simulink model "multi__micro1primarysecondarynn"  (R2015a)
settings: Solver=ode23tb  StartTime=0.0  StopTime=2
model workspace: external: MAT-File D:\google drive\project\nn1\matla.mat (data not in the file)
undefined symbols (not defined in the file): cf, gam, gamp, k1, k2, k3, k5, Lc, lf, mp1, mp2, Mu, nq1, nq2, rc, sig, sigp, td, wn
libraries: powerlib x115, powerlib_meascontrol x32, powerlib_extras x2
(part 1 of 3)
settings Model: Creator=David  LastModifiedBy=David
settings SolverCC: ZeroCrossControl=DisableAll  ZeroCrossAlgorithm=Adaptive  AlgebraicLoopSolver=LineSearch
settings DataIOCC: LimitDataPoints=off  SaveFormat=StructureWithTime  SaveOutput=off  SignalLogging=off  SaveTime=off
settings OptimizationCC: EfficientMapNaN2IntZero=off  SimCompilerOptimization=on
settings DebuggingCC: MaxConsecutiveZCsMsg=none
settings HardwareCC: TargetLongLongMode=on  TargetIntDivRoundTo=Zero  TargetEndianess=LittleEndian  TargetHWDeviceType=MATLAB Host  ProdEqTarget=off
settings CodeAppCC: MaxIdLength=128
settings GRTTargetCC: CombineOutputUpdateFcns=off  GRTInterface=on  RTWCAPISignals=on

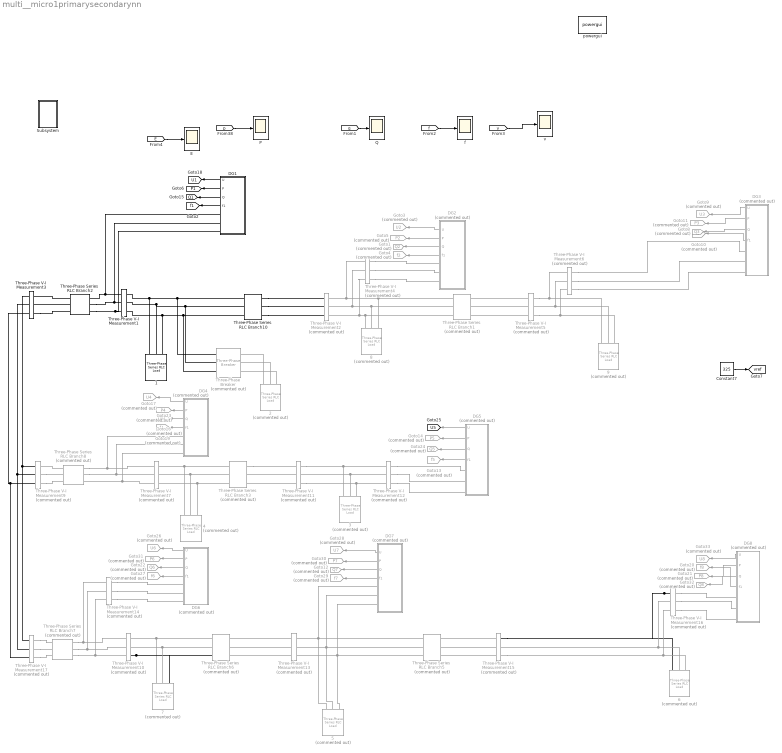
== system multi__micro1primarysecondarynn ==
  "  1" : powerlib/Elements/Three-Phase Series RLC Load  LConnTagsString=A|B|C  Configuration=Y (grounded)  NominalVoltage=vrms  NominalFrequency=50  ActivePower=18.5e3  InductivePower=14e3  CapacitivePower=0  Measurements=None  LoadType=constant Z
  "  2" : powerlib/Elements/Three-Phase Series RLC Load  Commented=on  LConnTagsString=A|B|C  Configuration=Y (grounded)  NominalVoltage=vrms  NominalFrequency=50  ActivePower=18.5e3  InductivePower=14e3  CapacitivePower=0  Measurements=None  LoadType=constant Z
  "  3" : powerlib/Elements/Three-Phase Series RLC Load  Commented=on  LConnTagsString=A|B|C  Configuration=Y (grounded)  NominalVoltage=vrms  NominalFrequency=50  ActivePower=16e3  InductivePower=11e3  CapacitivePower=0  Measurements=None  LoadType=constant Z
  "  4" : powerlib/Elements/Three-Phase Series RLC Load  Commented=on  LConnTagsString=A|B|C  Configuration=Y (grounded)  NominalVoltage=vrms  NominalFrequency=50  ActivePower=18.5e3  InductivePower=14e3  CapacitivePower=0  Measurements=None  LoadType=constant Z
  "  5" : powerlib/Elements/Three-Phase Series RLC Load  Commented=on  LConnTagsString=A|B|C  Configuration=Y (grounded)  NominalVoltage=vrms  NominalFrequency=50  ActivePower=15.3e3  InductivePower=10e3  CapacitivePower=0  Measurements=None  LoadType=constant Z
  "  6" : powerlib/Elements/Three-Phase Series RLC Load  Commented=on  LConnTagsString=A|B|C  Configuration=Y (grounded)  NominalVoltage=vrms  NominalFrequency=50  ActivePower=15.6e3  InductivePower=9.6e3  CapacitivePower=0  Measurements=None  LoadType=constant Z
  "  7" : powerlib/Elements/Three-Phase Series RLC Load  Commented=on  LConnTagsString=A|B|C  Configuration=Y (grounded)  NominalVoltage=vrms  NominalFrequency=50  ActivePower=20e3  InductivePower=15e3  CapacitivePower=0  Measurements=None  LoadType=constant Z
  "  8" : powerlib/Elements/Three-Phase Series RLC Load  Commented=on  LConnTagsString=A|B|C  Configuration=Y (grounded)  NominalVoltage=vrms  NominalFrequency=50  ActivePower=15e3  InductivePower=12e3  CapacitivePower=0  Measurements=None  LoadType=constant Z
  "  9" : powerlib/Elements/Three-Phase Series RLC Load  Commented=on  LConnTagsString=A|B|C  Configuration=Y (grounded)  NominalVoltage=vrms  NominalFrequency=50  ActivePower=12e3  InductivePower=8e3  CapacitivePower=0  Measurements=None  LoadType=constant Z
  Constant7 : Constant  Value=325
  DG1 : Subsystem
  DG2 : Subsystem  Commented=on
  DG3 : Subsystem  Commented=on
  DG4 : Subsystem  Commented=on
  DG5 : Subsystem  Commented=on
  DG6 : Subsystem  Commented=on
  DG7 : Subsystem  Commented=on
  DG8 : Subsystem  Commented=on
  E : Scope
      settings: TimeRange=0.03351610580764283  YMin=-1.5  YMax=-0.1  SaveName=E
  Goto1 : Goto  Commented=on  GotoTag=Q2  TagVisibility=global
  Goto10 : Goto  Commented=on  GotoTag=f3  TagVisibility=global
  Goto11 : Goto  Commented=on  GotoTag=P3  TagVisibility=global
  Goto12 : Goto  Commented=on  GotoTag=Q7  TagVisibility=global
  Goto13 : Goto  Commented=on  GotoTag=f5  TagVisibility=global
  Goto14 : Goto  Commented=on  GotoTag=P5  TagVisibility=global
  Goto16 : Goto  Commented=on  GotoTag=Q4  TagVisibility=global
  Goto17 : Goto  Commented=on  GotoTag=U4  TagVisibility=global
  Goto19 : Goto  Commented=on  GotoTag=f4  TagVisibility=global
  Goto20 : Goto  Commented=on  GotoTag=f8  TagVisibility=global
  Goto21 : Goto  Commented=on  GotoTag=P8  TagVisibility=global
  Goto22 : Goto  Commented=on  GotoTag=Q6  TagVisibility=global
  Goto23 : Goto  Commented=on  GotoTag=P4  TagVisibility=global
  Goto24 : Goto  Commented=on  GotoTag=Q5  TagVisibility=global
  Goto26 : Goto  Commented=on  GotoTag=U6  TagVisibility=global
  Goto27 : Goto  Commented=on  GotoTag=f6  TagVisibility=global
  Goto28 : Goto  Commented=on  GotoTag=U7  TagVisibility=global
  Goto29 : Goto  Commented=on  GotoTag=f7  TagVisibility=global
  Goto3 : Goto  Commented=on  GotoTag=U2  TagVisibility=global
  Goto30 : Goto  Commented=on  GotoTag=P7  TagVisibility=global
  Goto31 : Goto  Commented=on  GotoTag=P6  TagVisibility=global
  Goto32 : Goto  Commented=on  GotoTag=Q8  TagVisibility=global
  Goto33 : Goto  Commented=on  GotoTag=U8  TagVisibility=global
  Goto4 : Goto  Commented=on  GotoTag=f2  TagVisibility=global
  Goto5 : Goto  Commented=on  GotoTag=P2  TagVisibility=global
  Goto8 : Goto  Commented=on  GotoTag=Q3  TagVisibility=global
  Goto9 : Goto  Commented=on  GotoTag=U3  TagVisibility=global
  P : Scope
      settings: TimeRange=0.8  YMin=-20000  YMax=110000  SaveName=P1
  Q : Scope
      settings: TimeRange=2  YMin=0  YMax=13000  SaveName=Q1
  Subsystem : Subsystem
  Three-Phase Series RLC Branch1 : powerlib/Elements/Three-Phase Series RLC Branch  Commented=on  LConnTagsString=A|B|C  RConnTagsString=A|B|C  BranchType=RL  Resistance=0.35  Inductance=0.68e-3  Capacitance=1e-6  Measurements=None
  Three-Phase Series RLC Branch10 : powerlib/Elements/Three-Phase Series RLC Branch  LConnTagsString=A|B|C  RConnTagsString=A|B|C  BranchType=RL  Resistance=0.23  Inductance=0.35e-3  Capacitance=1e-6  Measurements=None
  Three-Phase Series RLC Branch2 : powerlib/Elements/Three-Phase Series RLC Branch  LConnTagsString=A|B|C  RConnTagsString=A|B|C  BranchType=RL  Resistance=0.195  Inductance=0.511e-3  Capacitance=1e-6  Measurements=None
  Three-Phase Series RLC Branch3 : powerlib/Elements/Three-Phase Series RLC Branch  Commented=on  LConnTagsString=A|B|C  RConnTagsString=A|B|C  BranchType=RL  Resistance=0.493  Inductance=0.494e-3  Capacitance=1e-6  Measurements=None
  Three-Phase Series RLC Branch5 : powerlib/Elements/Three-Phase Series RLC Branch  Commented=on  LConnTagsString=A|B|C  RConnTagsString=A|B|C  BranchType=RL  Resistance=0.161  Inductance=0.372e-3  Capacitance=1e-6  Measurements=None
  Three-Phase Series RLC Branch6 : powerlib/Elements/Three-Phase Series RLC Branch  Commented=on  LConnTagsString=A|B|C  RConnTagsString=A|B|C  BranchType=RL  Resistance=0.1  Inductance=0.318e-3  Capacitance=1e-6  Measurements=None
  Three-Phase Series RLC Branch7 : powerlib/Elements/Three-Phase Series RLC Branch  Commented=on  LConnTagsString=A|B|C  RConnTagsString=A|B|C  BranchType=RL  Resistance=0.1  Inductance=0.318e-3  Capacitance=1e-6  Measurements=None
  Three-Phase Series RLC Branch8 : powerlib/Elements/Three-Phase Series RLC Branch  Commented=on  LConnTagsString=A|B|C  RConnTagsString=A|B|C  BranchType=RL  Resistance=0.25  Inductance=0.375e-3  Capacitance=1e-6  Measurements=None
  Three-Phase V-I Measurement1 : powerlib/Measurements/Three-Phase V-I Measurement  VoltageMeasurement=no  SetLabelV=off  LabelV=Va  Vpu=off  VpuLL=off  CurrentMeasurement=no  SetLabelI=off  LabelI=Iabc  Ipu=off  Pbase=100e6  Vbase=500e3  OutputType=Complex  PhasorSimulation=off  PSBequivalent=0
  Three-Phase V-I Measurement{2,4..7,9..17} (14 alike) : powerlib/Measurements/Three-Phase V-I Measurement  Commented=on  VoltageMeasurement=no  SetLabelV=off  LabelV=Va  Vpu=off  VpuLL=off  CurrentMeasurement=no  SetLabelI=off  LabelI=Iabc  Ipu=off  Pbase=100e6  Vbase=500e3  OutputType=Complex  PhasorSimulation=off  PSBequivalent=0
  Three-Phase V-I Measurement3 : powerlib/Measurements/Three-Phase V-I Measurement  VoltageMeasurement=no  SetLabelV=off  LabelV=Va  Vpu=off  VpuLL=off  CurrentMeasurement=no  SetLabelI=off  LabelI=Iabc  Ipu=off  Pbase=100e6  Vbase=500e3  OutputType=Complex  PhasorSimulation=off  PSBequivalent=0
  Three-Phase Breaker : powerlib/Elements/Three-Phase Breaker  Commented=on  InitialState=open  SwitchA=on  SwitchB=on  SwitchC=on  SwitchTimes=0.5  External=off  BreakerResistance=0.01  SnubberResistance=1e6  SnubberCapacitance=inf  Measurements=None
  f : Scope
      settings: TimeRange=1  YMin=0  YMax=50  SaveName=f1
  powergui : powerlib/powergui  Priority=1  SimulationMode=Discrete  SolverType=Tustin/Backward Euler (TBE)  SampleTime=5e-5  frequency=50  SPID=off  DisableSnubberDevices=off  DisableRonSwitches=off  DisableVfSwitches=off  SwTol=0  DisplayEquations=off  Interpol=off  methode=off  Ts=100  FunctionMessages=off  echomessages=off  HookPort=off  EnableUseOfTLC=off  x0status=blocks  frequencyindice=0  Pbase=100e6  ErrMax=1e-4  Iterations=50  UnitsV=kV  UnitsW=MW  buscounter=0  RestoreLinks=warning  ResistiveCurrentMeasurement=off  Frange=[0:2:500]  Ylog=off  Xlog=on  ShowGrid=off  save=off  variable=ZData  structure=0  ZoomFFT=off  StartTime=0.0  cycles=1  DisplayStyle=1  fundamental=60  FreqAxis=off  MaxFrequency=1000  frequencyindicesteady=1  RmsSteady=1  display=off
  v : Scope
      settings: TimeRange=0.1127673055614255  YMin=2.77556e-17  YMax=1  SaveName=v1
  tag scope: P1=global, Q1=global, U1=global, U5=global, f1=global, vref=global
  wires:
  Constant7/1 -> [vref]
  DG2/1(U) -> Goto3/1
  DG2/3(Q) -> Goto1/1
  DG2/2(P) -> Goto5/1
  DG2/4(f1) -> Goto4/1
  DG4/3(Q) -> Goto16/1
  DG4/2(P) -> Goto23/1
  DG4/4(f1) -> Goto19/1
  DG5/1(U) -> [U5]
  DG5/4(f1) -> Goto13/1
  DG5/2(P) -> Goto14/1
  DG5/3(Q) -> Goto24/1
  DG8/1(U) -> Goto33/1
  DG8/4(f1) -> Goto20/1
  DG8/2(P) -> Goto21/1
  DG8/3(Q) -> Goto32/1
  [p] -> P/1
  [q] -> Q/1
  [f] -> f/1
  [v] -> v/1
  DG3/1(U) -> Goto9/1
  DG3/4(f1) -> Goto10/1
  DG3/2(P) -> Goto11/1
  DG3/3(Q) -> Goto8/1
  DG6/3(Q) -> Goto22/1
  DG6/2(P) -> Goto31/1
  DG6/4(f1) -> Goto27/1
  DG6/1(U) -> Goto26/1
  DG7/1(U) -> Goto28/1
  DG7/3(Q) -> Goto12/1
  DG7/2(P) -> Goto30/1
  DG7/4(f1) -> Goto29/1
  [E] -> E/1
  DG4/1(U) -> Goto17/1
  DG1/3(Q) -> [Q1]
  DG1/2(P) -> [P1]
  DG1/1(U) -> [U1]
  DG1/4(f1) -> [f1]
  connections:
  Three-Phase Series RLC Branch1/LConn1 -- Three-Phase V-I Measurement4/LConn1 -- Three-Phase V-I Measurement2/RConn1 -- "  8"/LConn3
  Three-Phase V-I Measurement5/RConn1 -- "  9"/LConn1 -- Three-Phase V-I Measurement6/LConn1
  Three-Phase V-I Measurement5/LConn1 -- Three-Phase Series RLC Branch1/RConn1
  Three-Phase V-I Measurement5/RConn3 -- "  9"/LConn3 -- Three-Phase V-I Measurement6/LConn3
  Three-Phase V-I Measurement6/LConn2 -- "  9"/LConn2 -- Three-Phase V-I Measurement5/RConn2
  Three-Phase Series RLC Branch10/LConn1 -- Three-Phase Breaker/LConn1 -- Three-Phase V-I Measurement1/RConn1 -- "  1"/LConn1
  Three-Phase Series RLC Branch10/LConn3 -- Three-Phase Breaker/LConn3 -- Three-Phase V-I Measurement1/RConn3 -- "  1"/LConn3
  Three-Phase Series RLC Branch10/LConn2 -- Three-Phase V-I Measurement1/RConn2 -- "  1"/LConn2 -- Three-Phase Breaker/LConn2
  Three-Phase V-I Measurement5/LConn2 -- Three-Phase Series RLC Branch1/RConn2
  Three-Phase V-I Measurement5/LConn3 -- Three-Phase Series RLC Branch1/RConn3
  "  3"/LConn1 -- Three-Phase V-I Measurement11/RConn1 -- Three-Phase V-I Measurement12/LConn1
  Three-Phase V-I Measurement11/RConn3 -- "  3"/LConn3 -- Three-Phase V-I Measurement12/LConn3
  Three-Phase V-I Measurement12/LConn2 -- Three-Phase V-I Measurement11/RConn2 -- "  3"/LConn2
  Three-Phase Series RLC Branch3/RConn1 -- Three-Phase V-I Measurement11/LConn1
  Three-Phase V-I Measurement11/LConn3 -- Three-Phase Series RLC Branch3/RConn3
  Three-Phase V-I Measurement11/LConn2 -- Three-Phase Series RLC Branch3/RConn2
  Three-Phase V-I Measurement16/LConn1 -- Three-Phase V-I Measurement15/RConn1 -- "  6"/LConn1
  Three-Phase V-I Measurement15/RConn3 -- "  6"/LConn3 -- Three-Phase V-I Measurement16/LConn3
  Three-Phase V-I Measurement16/LConn2 -- "  6"/LConn2 -- Three-Phase V-I Measurement15/RConn2
  Three-Phase Series RLC Branch6/LConn1 -- "  7"/LConn1 -- Three-Phase V-I Measurement10/RConn1
  Three-Phase V-I Measurement10/RConn3 -- Three-Phase Series RLC Branch6/LConn3 -- "  7"/LConn3
  Three-Phase Series RLC Branch6/LConn2 -- "  7"/LConn2 -- Three-Phase V-I Measurement10/RConn2
  Three-Phase V-I Measurement13/LConn2 -- Three-Phase Series RLC Branch6/RConn2
  Three-Phase V-I Measurement13/LConn3 -- Three-Phase Series RLC Branch6/RConn3
  Three-Phase V-I Measurement15/LConn1 -- Three-Phase Series RLC Branch5/RConn1
  Three-Phase V-I Measurement15/LConn2 -- Three-Phase Series RLC Branch5/RConn2
  Three-Phase V-I Measurement13/LConn1 -- Three-Phase Series RLC Branch6/RConn1
  Three-Phase V-I Measurement15/LConn3 -- Three-Phase Series RLC Branch5/RConn3
  Three-Phase Series RLC Branch7/LConn1 -- Three-Phase V-I Measurement14/LConn1 -- Three-Phase V-I Measurement10/LConn1
  Three-Phase Series RLC Branch7/LConn2 -- Three-Phase V-I Measurement14/LConn2 -- Three-Phase V-I Measurement10/LConn2
  Three-Phase Series RLC Branch7/LConn3 -- Three-Phase V-I Measurement14/LConn3 -- Three-Phase V-I Measurement10/LConn3
  Three-Phase V-I Measurement17/RConn1 -- Three-Phase Series RLC Branch7/RConn1
  Three-Phase V-I Measurement17/RConn2 -- Three-Phase Series RLC Branch7/RConn2
  Three-Phase V-I Measurement17/RConn3 -- Three-Phase Series RLC Branch7/RConn3
  Three-Phase Series RLC Branch8/RConn1 -- Three-Phase V-I Measurement9/RConn1
  Three-Phase V-I Measurement9/RConn2 -- Three-Phase Series RLC Branch8/RConn2
  Three-Phase V-I Measurement9/RConn3 -- Three-Phase Series RLC Branch8/RConn3
  Three-Phase V-I Measurement3/LConn1 -- Three-Phase V-I Measurement17/LConn1 -- Three-Phase V-I Measurement9/LConn1
  Three-Phase V-I Measurement3/LConn2 -- Three-Phase V-I Measurement17/LConn2 -- Three-Phase V-I Measurement9/LConn2
  Three-Phase V-I Measurement3/LConn3 -- Three-Phase V-I Measurement9/LConn3 -- Three-Phase V-I Measurement17/LConn3
  Three-Phase Series RLC Branch1/LConn3 -- Three-Phase V-I Measurement4/LConn3 -- Three-Phase V-I Measurement2/RConn3 -- "  8"/LConn1
  Three-Phase Series RLC Branch1/LConn2 -- Three-Phase V-I Measurement4/LConn2 -- Three-Phase V-I Measurement2/RConn2 -- "  8"/LConn2
  Three-Phase Series RLC Branch2/RConn2 -- Three-Phase V-I Measurement3/RConn2
  Three-Phase Series RLC Branch2/RConn1 -- Three-Phase V-I Measurement3/RConn1
  Three-Phase V-I Measurement3/RConn3 -- Three-Phase Series RLC Branch2/RConn3
  Three-Phase Series RLC Branch2/LConn2 -- DG1/RConn2 -- Three-Phase V-I Measurement1/LConn2
  Three-Phase Series RLC Branch2/LConn3 -- DG1/RConn3 -- Three-Phase V-I Measurement1/LConn3
  Three-Phase V-I Measurement1/LConn1 -- DG1/RConn1 -- Three-Phase Series RLC Branch2/LConn1
  Three-Phase V-I Measurement4/RConn1 -- DG2/RConn1
  Three-Phase V-I Measurement4/RConn2 -- DG2/RConn2
  Three-Phase V-I Measurement4/RConn3 -- DG2/RConn3
  Three-Phase V-I Measurement6/RConn1 -- DG3/RConn1
  Three-Phase V-I Measurement6/RConn2 -- DG3/RConn2
  Three-Phase V-I Measurement6/RConn3 -- DG3/RConn3
  Three-Phase Series RLC Branch8/LConn1 -- DG4/RConn1 -- Three-Phase V-I Measurement7/LConn1
  Three-Phase Series RLC Branch8/LConn2 -- DG4/RConn2 -- Three-Phase V-I Measurement7/LConn2
  Three-Phase V-I Measurement7/LConn3 -- DG4/RConn3 -- Three-Phase Series RLC Branch8/LConn3
  Three-Phase V-I Measurement12/RConn1 -- DG5/RConn1
  Three-Phase V-I Measurement12/RConn2 -- DG5/RConn2
  Three-Phase V-I Measurement12/RConn3 -- DG5/RConn3
  Three-Phase V-I Measurement14/RConn1 -- DG6/RConn1
  Three-Phase V-I Measurement14/RConn2 -- DG6/RConn2
  Three-Phase V-I Measurement14/RConn3 -- DG6/RConn3
  Three-Phase Series RLC Branch5/LConn1 -- DG7/RConn1 -- "  5"/LConn1 -- Three-Phase V-I Measurement13/RConn1
  Three-Phase Series RLC Branch5/LConn2 -- DG7/RConn2 -- "  5"/LConn2 -- Three-Phase V-I Measurement13/RConn2
  Three-Phase Series RLC Branch5/LConn3 -- DG7/RConn3 -- "  5"/LConn3 -- Three-Phase V-I Measurement13/RConn3
  Three-Phase V-I Measurement16/RConn2 -- DG8/RConn2
  Three-Phase V-I Measurement16/RConn1 -- DG8/RConn1
  Three-Phase V-I Measurement16/RConn3 -- DG8/RConn3
  Three-Phase Series RLC Branch3/LConn1 -- "  4"/LConn1 -- Three-Phase V-I Measurement7/RConn1
  Three-Phase Series RLC Branch3/LConn2 -- "  4"/LConn2 -- Three-Phase V-I Measurement7/RConn2
  Three-Phase Series RLC Branch3/LConn3 -- "  4"/LConn3 -- Three-Phase V-I Measurement7/RConn3
  "  2"/LConn1 -- Three-Phase Breaker/RConn1
  "  2"/LConn2 -- Three-Phase Breaker/RConn2
  "  2"/LConn3 -- Three-Phase Breaker/RConn3
  Three-Phase Series RLC Branch10/RConn1 -- Three-Phase V-I Measurement2/LConn1
  Three-Phase Series RLC Branch10/RConn2 -- Three-Phase V-I Measurement2/LConn2
  Three-Phase Series RLC Branch10/RConn3 -- Three-Phase V-I Measurement2/LConn3

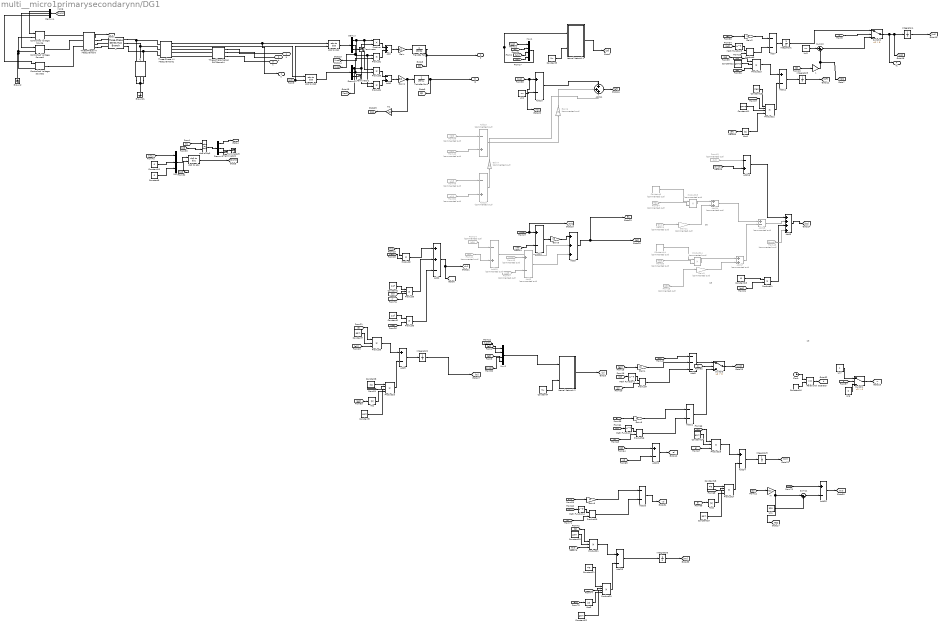
== system multi__micro1primarysecondarynn/DG1 ==
  note: SE
  note: SE
  note: SE
  Abs{,1..3} (4 alike) : Abs
  Add : Sum
  Add1 : Sum  Inputs=-+
  Add{4,9..10,12,22,24..26} (8 alike) : Sum  Inputs=+-
  Add11 : Sum  Inputs=+++
  Add13 : Sum  Commented=on  Inputs=-+
  Add14 : Sum  Commented=on
  Add15 : Sum  Commented=on  Inputs=-+
  Add16 : Sum  Inputs=-+
  Add17 : Sum  Commented=on
  Add18 : Sum  Commented=on  Inputs=+-
  Add19 : Sum  Commented=on  Inputs=-+
  Add2 : Sum  Inputs=++-
  Add20 : Sum  Inputs=--
  Add21 : Sum  Inputs=--
  Add3 : Sum  Inputs=+++
  Add5 : Sum  Inputs=++++
  Add6 : Sum  Commented=on  Inputs=+-
  Add7 : Sum  Inputs=--
  Add8 : Sum  Inputs=---
  C : powerlib/Elements/Three-Phase Series RLC Branch  LConnTagsString=A|B|C  RConnTagsString=A|B|C  BranchType=C  Resistance=1  Inductance=1e-3  Capacitance=cf  Measurements=None
  Clock : Clock
  Constant1 : Constant  Value=1/cf
  Constant10 : Constant  Value=0
  Constant11 : Constant  Value=gamp
  Constant12 : Constant  Value=gamp
  Constant13 : Constant  Value=sigp
  Constant14 : Constant  Commented=on  Value=-31.446
  Constant15 : Constant  Value=k1
  Constant16 : Constant  Value=0.05
  Constant{7,9,17,19..20,22} (6 alike) : Constant  Value=gam
  Constant18 : Constant  Value=sig
  Constant2 : Constant  Value=1/cf
  Constant21 : Constant  Value=sig
  Constant3 : Constant  Value=Mu
  Constant4 : Constant  Value=Mu
  Constant5 : Constant  Commented=on  Value=-31.446
  Constant6 : Constant  Value=0
  Constant8 : Constant  Value=sig
  Controlled Voltage Source : powerlib/Electrical Sources/Controlled Voltage Source  Initialize=on  Source_Type=AC  Amplitude=0  Phase=0  Frequency=0  Measurements=None
  Controlled Voltage Source1 : powerlib/Electrical Sources/Controlled Voltage Source  Initialize=on  Source_Type=AC  Amplitude=0  Phase=0  Frequency=0  Measurements=None
  Controlled Voltage Source2 : powerlib/Electrical Sources/Controlled Voltage Source  Initialize=on  Source_Type=AC  Amplitude=0  Phase=0  Frequency=0  Measurements=None
  Demux{,1,3..4} (4 alike) : Demux  Outputs=3
  From13 : From  Commented=on  GotoTag=Q11  TagVisibility=global
  From14 : From  Commented=on  GotoTag=NQ8
  From25 : From  Commented=on  GotoTag=Q88  TagVisibility=global
  From39 : From  Commented=on  GotoTag=MP8  TagVisibility=global
  From40 : From  Commented=on  GotoTag=MP2  TagVisibility=global
  From41 : From  Commented=on  GotoTag=NQ2  TagVisibility=global
  From43 : From  Commented=on  GotoTag=dv8  TagVisibility=global
  From46 : From  Commented=on  GotoTag=vod
  From47 : From  Commented=on  GotoTag=vod8
  From48 : From  Commented=on  GotoTag=dvodi
  From49 : From  Commented=on  GotoTag=w18  TagVisibility=global
  From52 : From  Commented=on  GotoTag=w11  TagVisibility=global
  From54 : From  Commented=on  GotoTag=NQ2  TagVisibility=global
  From55 : From  Commented=on  GotoTag=NQ8  TagVisibility=global
  Gain : Gain  Gain=3/2
  Gain1 : Gain  Gain=3/2
  Gain11 : Gain  Commented=on  Gain=31.446
  Gain2 : Gain  Gain=k3
  Gain3 : Gain  Commented=on  Gain=31.446
  Gain4 : Gain  Gain=k2
  Gain5 : Gain  Gain=k5
  Gain6 : Gain  Commented=on  Gain=k5
  Gain7 : Gain  Commented=on  Gain=k5
  Gain8 : Gain  Gain=k2
  Gain9 : Gain  Gain=k2
  Ground : powerlib/Elements/Ground  LConnTagsString=a
  Ground1 : powerlib/Elements/Ground  LConnTagsString=a
  Integrator1 : Integrator  UpperSaturationLimit=321  LowerSaturationLimit=314.16
  Integrator{2..3,5..6} (4 alike) : Integrator  InitialCondition=zeros(16,1)  UpperSaturationLimit=314.16  ZeroCross=off
  Integrator4 : Integrator  UpperSaturationLimit=314.16  ZeroCross=off
  L : powerlib/Elements/Three-Phase Series RLC Branch  LConnTagsString=A|B|C  RConnTagsString=A|B|C  BranchType=RL  Resistance=0.1  Inductance=lf  Capacitance=1e-6  Measurements=None
  Math Function{1..4} (4 alike) : Math  Operator=transpose  OutputSignalType=real  SaturateOnIntegerOverflow=on
  Mux : Mux  Inputs=3
  Mux1 : Mux
  Mux2 : Mux
  Neural Network 1 : MATLAB Function  TreatAsAtomicUnit=on
  Neural Network 2 : MATLAB Function  TreatAsAtomicUnit=on
  Product{,1,3..4} (4 alike) : Product  RndMeth=Zero
  Product{10,12,17,20} (4 alike) : Product  Inputs=4
  Product11 : Product
  Product{5,8,13,18,21} (5 alike) : Product  Inputs=3
  Product14 : Product  Commented=on
  Product15 : Product  Commented=on
  Product{7,9,16,19} (4 alike) : Product  Multiplication=Matrix(*)
  Product2 : Product
  Product6 : Product
  Relational Operator : RelationalOperator  InputSameDT=on
  Sum10 : Sum  Inputs=|+-
  Sum11 : Sum  Inputs=|-+
  Switch1 : Switch  Criteria=u2 > Threshold
  Switch2 : Switch  Criteria=u2 > Threshold
  Switch3 : Switch  Criteria=u2 > Threshold
  Terminator{,1..3} (4 alike) : Terminator
  Three-Phase Series RLC Branch4 : powerlib/Elements/Three-Phase Series RLC Branch  LConnTagsString=A|B|C  RConnTagsString=A|B|C  BranchType=RL  Resistance=rc  Inductance=Lc  Capacitance=1e-6  Measurements=None
  Three-Phase V-I Measurement : powerlib/Measurements/Three-Phase V-I Measurement  VoltageMeasurement=phase-to-ground  SetLabelV=off  LabelV=Vabc  Vpu=off  VpuLL=off  CurrentMeasurement=yes  SetLabelI=off  LabelI=Iabc  Ipu=off  Pbase=100e6  Vbase=500e3  OutputType=Complex  PhasorSimulation=off  PSBequivalent=0
  Three-Phase V-I Measurement1 : powerlib/Measurements/Three-Phase V-I Measurement  VoltageMeasurement=phase-to-ground  SetLabelV=off  LabelV=Vabc  Vpu=off  VpuLL=off  CurrentMeasurement=yes  SetLabelI=off  LabelI=Iabc  Ipu=off  Pbase=100e6  Vbase=500e3  OutputType=Complex  PhasorSimulation=off  PSBequivalent=0
  Transfer Fcn : TransferFcn  Denominator=[td 1]
  Transfer Fcn1 : TransferFcn  Denominator=[td 1]
  Un1 : Constant  Value=325
  Un2 : Constant  Value=wn
  Un3 : Constant  Value=wn
  Un6 : Constant  Value=0
  Un7 : Constant
  abc to dq0 : powerlib_meascontrol/Transformations/abc to dq0  Alignment=90 degrees behind phase A axis
  abc to dq1 : powerlib_meascontrol/Transformations/abc to dq0  Alignment=90 degrees behind phase A axis
  abc to dq3 : powerlib_meascontrol/Transformations/abc to dq0  Alignment=90 degrees behind phase A axis
  dq0 to abc : powerlib_meascontrol/Transformations/dq0 to abc  Alignment=90 degrees behind phase A axis
  m : Gain  Gain=nq1
  m1 : Gain  Gain=nq1
  n : Gain  Gain=mp1
  a : PMIOPort  Tag=PMCPort  Port=1  Side=Right
  b : PMIOPort  Tag=PMCPort  Port=2  Side=Right
  c : PMIOPort  Tag=PMCPort  Port=3  Side=Right
  U : Outport
  P : Outport  Port=2
  Q : Outport  Port=3
  f1 : Outport  Port=4
  tag scope: E1=global, MP2=global, NQ2=global, Q11=global, dv1=global, el=global, evd=global, rr=global, ti=global, vd=global, vod1=global, w11=global
  wires:
  [PWM] -> Demux4/1
  Three-Phase V-I Measurement1/1 -> U/1, abc to dq1/1
  Demux/1 -> [vod], Product/1, Product3/1
  Demux1/1 -> [iod], Product/2, Product4/1
  Demux/2 -> [voq], Product1/1, Product4/2
  Demux1/2 -> Product1/2, Product3/2
  Product/1 -> Add/1
  Product1/1 -> Add/2
  Product3/1 -> Add1/1
  Product4/1 -> Add1/2
  [wt] -> abc to dq1/2, abc to dq0/2
  Demux4/1 -> Controlled Voltage Source/1
  Demux4/2 -> Controlled Voltage Source1/1
  Demux4/3 -> Controlled Voltage Source2/1
  Three-Phase V-I Measurement/2 -> [IL]
  Add/1 -> Gain/1
  Gain/1 -> Transfer Fcn/1
  Add1/1 -> Gain1/1
  Gain1/1 -> m1/1, Transfer Fcn1/1
  abc to dq1/1 -> Demux/1
  abc to dq0/1 -> Demux1/1
  Demux/3 -> Terminator/1
  Demux1/3 -> Terminator1/1
  [vod] -> [vod1], Add4/1
  Gain4/1 -> Add8/2
  [e2] -> Gain4/1
  [S] -> Product7/2
  [W] -> Math Function1/1
  Math Function1/1 -> Product7/1
  Product7/1 -> Add8/3
  [S] -> Product8/1
  Constant7/1 -> Product8/2
  [e2] -> Product8/3
  Product8/1 -> Add9/1
  Constant8/1 -> Product10/1
  [W] -> Product10/2
  Product10/1 -> Add9/2
  Constant9/1 -> Product10/3
  Add9/1 -> Integrator2/1
  [vref] -> Add4/2
  [IL] -> abc to dq3/1
  Demux3/1 -> [Id]
  Demux3/2 -> Terminator3/1
  [wt] -> abc to dq3/2
  Mux/1 -> dq0 to abc/1
  [wt] -> dq0 to abc/2
  abc to dq3/1 -> Demux3/1
  dq0 to abc/1 -> [PWM]
  Demux3/3 -> Terminator2/1
  [vn1] -> Mux/1
  Constant10/1 -> Mux/2
  Constant6/1 -> Mux/3
  Transfer Fcn/1 -> P/1, [P]
  Transfer Fcn1/1 -> Q/1, [Q]
  [w1] -> Mux1/1
  [ef] -> Mux1/2
  [w1] -> Mux1/3
  [MP2] -> Mux1/4
  [w1] -> [w11], Add10/1
  Un2/1 -> Add10/2
  [Sf] -> Product13/1
  Constant12/1 -> Product13/2
  [ef] -> Product13/3
  Product13/1 -> Add12/1
  Constant13/1 -> Product12/1
  [Wf] -> Product12/2
  Product12/1 -> Add12/2
  Constant11/1 -> Product12/3
  Add12/1 -> Integrator3/1
  Integrator3/1 -> [Wf]
  Three-Phase V-I Measurement1/2 -> abc to dq0/1
  Add10/1 -> Add11/1
  From39/1 -> Add13/1
  From40/1 -> Add13/2
  Add13/1 -> Gain6/1
  Gain6/1 -> Add11/2
  From14/1 -> Add15/1
  From41/1 -> Add15/2
  Add15/1 -> Add3/2
  [e1] -> Add8/1
  Add4/1 -> Gain5/1
  Gain5/1 -> Add3/1
  [vod] -> Mux2/1
  [e1] -> Mux2/2
  [dvodi] -> Mux2/3
  [e2] -> Mux2/4
  Constant5/1 -> Product15/1
  From54/1 -> Product15/2
  Product15/1 -> Add14/1
  From13/1 -> Gain11/1
  Constant14/1 -> Product14/1
  From55/1 -> Product14/2
  Product14/1 -> Add17/1
  From25/1 -> Gain3/1
  Add17/1 -> Add18/2
  Add14/1 -> Add18/1
  Gain3/1 -> Add17/2
  Gain11/1 -> Add14/2
  Add18/1 -> Add5/2
  Constant15/1 -> Product11/1
  [e1] -> Product11/2
  Product11/1 -> Add5/3
  From43/1 -> Add16/1
  Add16/1 -> Add5/1
  [dvodi] -> Add16/2
  From46/1 -> Add6/1
  From47/1 -> Add6/2
  Add6/1 -> Add3/3
  From48/1 -> Add5/4
  m1/1 -> [Q11]
  From49/1 -> Add19/1
  From52/1 -> Add19/2
  Add19/1 -> Gain7/1
  Gain7/1 -> Add11/3
  Neural Network 1/1(Sz1) -> [Sf]
  Abs/1 -> Product10/4
  [e2] -> Abs/1
  [ef] -> Gain2/1
  [Sf] -> Product9/2
  [Wf] -> Math Function3/1
  Math Function3/1 -> Product9/1
  Gain2/1 -> Add7/1
  Product9/1 -> Add7/2
  Add7/1 -> Integrator1/1
  Abs1/1 -> Product12/4
  [ef] -> Abs1/1
  Neural Network 2/1(Sz1) -> [S]
  Constant4/1 -> Neural Network 2/2(mu)
  Mux2/1 -> Neural Network 2/1(X)
  Constant3/1 -> Neural Network 1/2(mu)
  Mux1/1 -> Neural Network 1/1(X)
  [ti] -> Switch1/2
  Un6/1 -> Switch1/3
  Un7/1 -> Switch1/1
  Switch1/1 -> [rr]
  Constant16/1 -> Relational Operator/2
  Clock/1 -> Relational Operator/1
  Relational Operator/1 -> [ti]
  Add3/1 -> [E1], [e1]
  Add5/1 -> [e2]
  Integrator4/1 -> [wt]
  Add11/1 -> [ef]
  [ti] -> Switch3/2
  Add8/1 -> Switch3/1
  Switch3/1 -> [vn1]
  [el] -> Gain8/1
  [S] -> Product16/2
  [Wl] -> Math Function2/1
  Math Function2/1 -> Product16/1
  Product16/1 -> Add21/2
  Gain8/1 -> Add21/1
  Add21/1 -> Switch3/3
  [Id] -> Add22/1
  [vd] -> Add22/2
  Add22/1 -> [el]
  [S] -> Product18/1
  Constant17/1 -> Product18/2
  [el] -> Product18/3
  Product18/1 -> Add24/1
  Constant18/1 -> Product17/1
  [Wl] -> Product17/2
  Product17/1 -> Add24/2
  Constant19/1 -> Product17/3
  Add24/1 -> Integrator5/1
  Integrator5/1 -> [Wl]
  Abs2/1 -> Product17/4
  [el] -> Abs2/1
  [vod] -> Add25/1
  Add25/1 -> [evd]
  Sum11/1 -> Add25/2
  [Q] -> m/1
  Un1/1 -> Sum11/2
  m/1 -> [NQ2], Sum11/1
  [evd] -> Gain9/1
  [S] -> Product19/2
  [Wv] -> Math Function4/1
  Math Function4/1 -> Product19/1
  Product19/1 -> Add20/2
  Gain9/1 -> Add20/1
  Add20/1 -> [vd]
  [S] -> Product21/1
  Constant20/1 -> Product21/2
  [evd] -> Product21/3
  Product21/1 -> Add26/1
  Constant21/1 -> Product20/1
  [Wv] -> Product20/2
  Product20/1 -> Add26/2
  Constant22/1 -> Product20/3
  Abs3/1 -> Product20/4
  [evd] -> Abs3/1
  Add26/1 -> Integrator6/1
  Integrator6/1 -> [Wv]
  Integrator2/1 -> [W]
  [w1] -> Product2/1
  [voq] -> Product2/2
  Product2/1 -> Add2/1
  Constant1/1 -> Product5/1
  [Id] -> Product5/2
  Product5/1 -> Add2/2
  Constant2/1 -> Product6/1
  [iod] -> Product6/2
  Product6/1 -> Add2/3
  Add2/1 -> [dvodi], [dv1]
  [rr] -> Product5/3
  [P] -> n/1
  Un3/1 -> Sum10/1  "f"
  n/1 -> [MP2], Sum10/2
  Integrator1/1 -> Switch2/1
  Switch2/1 -> f1/1, [w1], Integrator4/1
  Sum10/1 -> Switch2/3
  [ti] -> Switch2/2
  connections:
  C/RConn1 -- Ground1/LConn1 -- C/RConn3 -- C/RConn2
  L/RConn2 -- Three-Phase V-I Measurement1/LConn2 -- C/LConn2
  L/RConn1 -- Three-Phase V-I Measurement1/LConn1 -- C/LConn1
  L/RConn3 -- Three-Phase V-I Measurement1/LConn3 -- C/LConn3
  Controlled Voltage Source/LConn1 -- Controlled Voltage Source1/LConn1 -- Ground/LConn1 -- Controlled Voltage Source2/LConn1
  Three-Phase V-I Measurement/LConn1 -- Controlled Voltage Source/RConn1
  Controlled Voltage Source1/RConn1 -- Three-Phase V-I Measurement/LConn2
  Controlled Voltage Source2/RConn1 -- Three-Phase V-I Measurement/LConn3
  Three-Phase V-I Measurement/RConn1 -- L/LConn1
  Three-Phase V-I Measurement/RConn2 -- L/LConn2
  Three-Phase V-I Measurement/RConn3 -- L/LConn3
  Three-Phase Series RLC Branch4/RConn1 -- Three-Phase V-I Measurement1/RConn1
  Three-Phase Series RLC Branch4/RConn2 -- Three-Phase V-I Measurement1/RConn2
  Three-Phase Series RLC Branch4/RConn3 -- Three-Phase V-I Measurement1/RConn3
  Three-Phase Series RLC Branch4/LConn3 -- c/RConn1
  Three-Phase Series RLC Branch4/LConn2 -- b/RConn1
  Three-Phase Series RLC Branch4/LConn1 -- a/RConn1

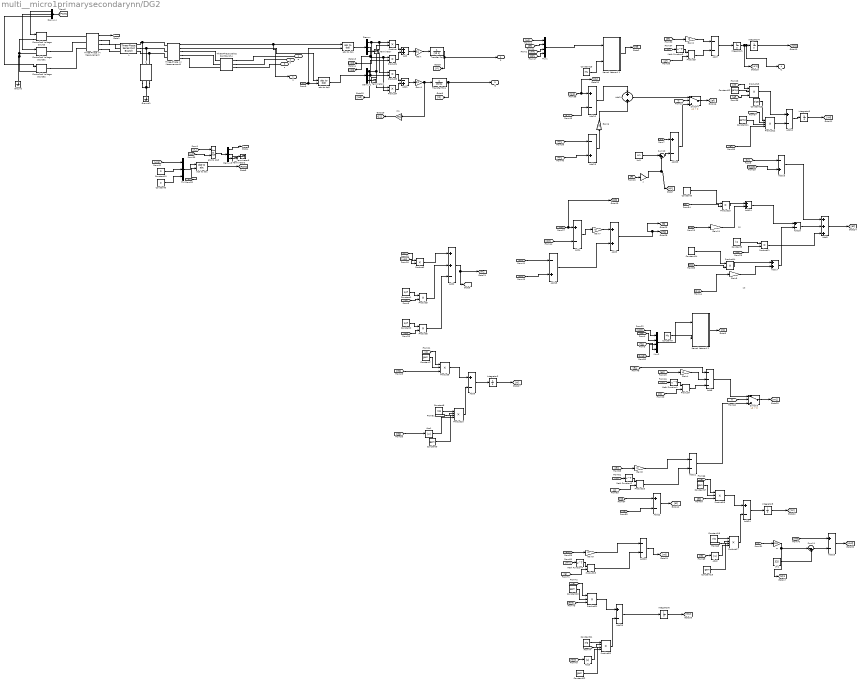
== system multi__micro1primarysecondarynn/DG2 ==
  note: SE
  note: SE
  Abs1 : Abs
  Abs2 : Abs
  Abs3 : Abs
  Add{,3,11,14,17} (5 alike) : Sum
  Add{1,13,15..16} (4 alike) : Sum  Inputs=-+
  Add{4,9..10,12,18,22..26} (10 alike) : Sum  Inputs=+-
  Add2 : Sum  Inputs=++-
  Add20 : Sum  Inputs=--
  Add21 : Sum  Inputs=--
  Add5 : Sum  Inputs=+++
  Add7 : Sum  Inputs=--
  Add8 : Sum  Inputs=---
  C : powerlib/Elements/Three-Phase Series RLC Branch  LConnTagsString=A|B|C  RConnTagsString=A|B|C  BranchType=C  Resistance=1  Inductance=1e-3  Capacitance=cf  Measurements=None
  Constant1 : Constant  Value=1/cf
  Constant10 : Constant  Value=0
  Constant11 : Constant  Value=gamp
  Constant12 : Constant  Value=gamp
  Constant13 : Constant  Value=sigp
  Constant14 : Constant  Value=-31.446
  Constant15 : Constant  Value=Mu
  Constant{7,9,17,19..20,22} (6 alike) : Constant  Value=gam
  Constant18 : Constant  Value=sig
  Constant2 : Constant  Value=1/cf
  Constant21 : Constant  Value=sig
  Constant3 : Constant  Value=-31.446
  Constant4 : Constant  Value=Mu
  Constant5 : Constant  Value=k1
  Constant6 : Constant  Value=0
  Constant8 : Constant  Value=sig
  Controlled Voltage Source : powerlib/Electrical Sources/Controlled Voltage Source  Initialize=on  Source_Type=AC  Amplitude=0  Phase=0  Frequency=0  Measurements=None
  Controlled Voltage Source1 : powerlib/Electrical Sources/Controlled Voltage Source  Initialize=on  Source_Type=AC  Amplitude=0  Phase=0  Frequency=0  Measurements=None
  Controlled Voltage Source2 : powerlib/Electrical Sources/Controlled Voltage Source  Initialize=on  Source_Type=AC  Amplitude=0  Phase=0  Frequency=0  Measurements=None
  Demux{,1,3..4} (4 alike) : Demux  Outputs=3
  Gain : Gain  Gain=3/2
  Gain1 : Gain  Gain=3/2
  Gain11 : Gain  Gain=31.446
  Gain2 : Gain  Gain=k3
  Gain4 : Gain  Gain=k2
  Gain5 : Gain  Gain=31.446
  Gain6 : Gain  Gain=k5
  Gain7 : Gain  Gain=k5
  Gain8 : Gain  Gain=k2
  Gain9 : Gain  Gain=k2
  Ground : powerlib/Elements/Ground  LConnTagsString=a
  Ground1 : powerlib/Elements/Ground  LConnTagsString=a
  Integrator1 : Integrator  UpperSaturationLimit=321  LowerSaturationLimit=314.16
  Integrator{2..3,5..6} (4 alike) : Integrator  InitialCondition=zeros(16,1)  UpperSaturationLimit=314.16  ZeroCross=off
  Integrator4 : Integrator  UpperSaturationLimit=314.16  ZeroCross=off
  L : powerlib/Elements/Three-Phase Series RLC Branch  LConnTagsString=A|B|C  RConnTagsString=A|B|C  BranchType=RL  Resistance=0.1  Inductance=lf  Capacitance=1e-6  Measurements=None
  Math Function{1..4} (4 alike) : Math  Operator=transpose  OutputSignalType=real  SaturateOnIntegerOverflow=on
  Mux : Mux  Inputs=3
  Mux1 : Mux
  Mux2 : Mux
  Neural Network 1 : MATLAB Function  TreatAsAtomicUnit=on
  Neural Network 2 : MATLAB Function  TreatAsAtomicUnit=on
  Product{,1,3..4} (4 alike) : Product  RndMeth=Zero
  Product{10,12,17,20} (4 alike) : Product  Inputs=4
  Product{2,5..6,11,14..15} (6 alike) : Product
  Product{8,13,18,21} (4 alike) : Product  Inputs=3
  Product{7,9,16,19} (4 alike) : Product  Multiplication=Matrix(*)
  Sum10 : Sum  Inputs=|+-
  Sum11 : Sum  Inputs=|-+
  Switch3 : Switch  Criteria=u2 > Threshold
  Switch4 : Switch  Criteria=u2 > Threshold
  Terminator{,1..3} (4 alike) : Terminator
  Three-Phase Series RLC Branch4 : powerlib/Elements/Three-Phase Series RLC Branch  LConnTagsString=A|B|C  RConnTagsString=A|B|C  BranchType=RL  Resistance=rc  Inductance=Lc  Capacitance=1e-6  Measurements=None
  Three-Phase V-I Measurement : powerlib/Measurements/Three-Phase V-I Measurement  VoltageMeasurement=no  SetLabelV=off  LabelV=Vabc  Vpu=off  VpuLL=off  CurrentMeasurement=yes  SetLabelI=off  LabelI=Iabc  Ipu=off  Pbase=100e6  Vbase=500e3  OutputType=Complex  PhasorSimulation=off  PSBequivalent=0
  Three-Phase V-I Measurement1 : powerlib/Measurements/Three-Phase V-I Measurement  VoltageMeasurement=phase-to-ground  SetLabelV=off  LabelV=Vabc  Vpu=off  VpuLL=off  CurrentMeasurement=yes  SetLabelI=off  LabelI=Iabc  Ipu=off  Pbase=100e6  Vbase=500e3  OutputType=Complex  PhasorSimulation=off  PSBequivalent=0
  Transfer Fcn : TransferFcn  Denominator=[td 1]
  Transfer Fcn1 : TransferFcn  Denominator=[td 1]
  Un1 : Constant  Value=325
  Un3 : Constant  Value=wn
  abc to dq0 : powerlib_meascontrol/Transformations/abc to dq0  Alignment=90 degrees behind phase A axis
  abc to dq1 : powerlib_meascontrol/Transformations/abc to dq0  Alignment=90 degrees behind phase A axis
  abc to dq3 : powerlib_meascontrol/Transformations/abc to dq0  Alignment=90 degrees behind phase A axis
  dq0 to abc : powerlib_meascontrol/Transformations/dq0 to abc  Alignment=90 degrees behind phase A axis
  m : Gain  Gain=nq1
  m1 : Gain  Gain=nq1
  n : Gain  Gain=mp1
  a : PMIOPort  Tag=PMCPort  Port=1  Side=Right
  b : PMIOPort  Tag=PMCPort  Port=2  Side=Right
  c : PMIOPort  Tag=PMCPort  Port=3  Side=Right
  U : Outport
  P : Outport  Port=2
  Q : Outport  Port=3
  f1 : Outport  Port=4
  tag scope: E2=global, MP1=global, NQ1=global, Q22=global, dv2=global, vod2=global, w12=global
  wires:
  [PWM] -> Demux4/1
  Three-Phase V-I Measurement1/1 -> U/1, abc to dq1/1
  Three-Phase V-I Measurement1/2 -> abc to dq0/1
  Demux/1 -> [vod], Product/1, Product3/1
  Demux1/1 -> [iod], Product/2, Product4/1
  Demux/2 -> [voq], Product1/1, Product4/2
  Demux1/2 -> Product1/2, Product3/2
  Product/1 -> Add/1
  Product1/1 -> Add/2
  Product3/1 -> Add1/1
  Product4/1 -> Add1/2
  [wt] -> abc to dq1/2, abc to dq0/2
  Demux4/1 -> Controlled Voltage Source/1
  Demux4/2 -> Controlled Voltage Source1/1
  Demux4/3 -> Controlled Voltage Source2/1
  Three-Phase V-I Measurement/1 -> [IL]
  Add/1 -> Gain/1
  Gain/1 -> Transfer Fcn/1
  Add1/1 -> Gain1/1
  Gain1/1 -> m1/1, Transfer Fcn1/1
  abc to dq1/1 -> Demux/1
  abc to dq0/1 -> Demux1/1
  [w1] -> Product2/1
  [voq] -> Product2/2
  Product2/1 -> Add2/1
  Constant1/1 -> Product5/1
  [Id] -> Product5/2
  Product5/1 -> Add2/2
  Constant2/1 -> Product6/1
  [iod] -> Product6/2
  Product6/1 -> Add2/3
  Add2/1 -> [dvodi], [dv2]
  Demux/3 -> Terminator/1
  Demux1/3 -> Terminator1/1
  Gain4/1 -> Add8/2
  [e2] -> Gain4/1
  [S] -> Product7/2
  [W] -> Math Function1/1
  Math Function1/1 -> Product7/1
  Product7/1 -> Add8/3
  [IL] -> abc to dq3/1
  Demux3/1 -> [Id]
  Demux3/2 -> Terminator3/1
  [wt] -> abc to dq3/2
  Mux/1 -> dq0 to abc/1
  [wt] -> dq0 to abc/2
  abc to dq3/1 -> Demux3/1
  dq0 to abc/1 -> [PWM]
  Demux3/3 -> Terminator2/1
  [vn1] -> Mux/1
  Constant10/1 -> Mux/2
  Constant6/1 -> Mux/3
  Transfer Fcn/1 -> P/1, [P]
  Transfer Fcn1/1 -> Q/1, [Q]
  [ef] -> Gain2/1
  [Sf] -> Product9/2
  [Wf] -> Math Function3/1
  Math Function3/1 -> Product9/1
  Gain2/1 -> Add7/1
  Product9/1 -> Add7/2
  [w1] -> Mux1/1
  [ef] -> Mux1/2
  [wn] -> Mux1/3
  [MP1] -> Mux1/4
  [w1] -> [w12], Add10/1
  [w11] -> Add10/2
  Add10/1 -> Add11/1
  [MP2] -> Add13/1
  [MP1] -> Add13/2
  Add13/1 -> Gain6/1
  [vod] -> [vod2], Add4/1
  [vod1] -> Add4/2
  Gain6/1 -> Add11/2
  [NQ2] -> Add15/1
  [NQ1] -> Add15/2
  [e1] -> Add8/1
  Add4/1 -> Gain7/1
  Add15/1 -> Add3/2
  Gain7/1 -> Add3/1
  [vod] -> Mux2/1
  [e1] -> Mux2/2
  [e2] -> Mux2/4
  [dvodi] -> Mux2/3
  Constant3/1 -> Product15/1
  [NQ1] -> Product15/2
  Product15/1 -> Add14/1
  [Q22] -> Gain11/1
  Constant14/1 -> Product14/1
  [NQ2] -> Product14/2
  Product14/1 -> Add17/1
  [Q11] -> Gain5/1
  Add17/1 -> Add18/2
  Add14/1 -> Add18/1
  Gain5/1 -> Add17/2
  Gain11/1 -> Add14/2
  Add18/1 -> Add5/2
  Constant5/1 -> Product11/1
  [e1] -> Product11/2
  Product11/1 -> Add5/3
  [dv1] -> Add16/1
  Add16/1 -> Add5/1
  [dvodi] -> Add16/2
  m1/1 -> [Q22]
  Neural Network 1/1(Sz1) -> [Sf]
  Neural Network 2/1(Sz1) -> [S]
  [S] -> Product8/1
  Constant7/1 -> Product8/2
  Product8/1 -> Add9/1
  Constant8/1 -> Product10/1
  [W] -> Product10/2
  Product10/1 -> Add9/2
  Constant9/1 -> Product10/3
  Add9/1 -> Integrator2/1
  Integrator2/1 -> [W]
  [e2] -> Abs1/1
  [Sf] -> Product13/1
  Constant12/1 -> Product13/2
  [ef] -> Product13/3
  Product13/1 -> Add12/1
  Constant13/1 -> Product12/1
  [Wf] -> Product12/2
  Product12/1 -> Add12/2
  Constant11/1 -> Product12/3
  Add12/1 -> Integrator3/1
  Integrator3/1 -> [Wf]
  [ef] -> Product12/4
  Constant4/1 -> Neural Network 2/2(mu)
  Mux2/1 -> Neural Network 2/1(X)
  Constant15/1 -> Neural Network 1/2(mu)
  Mux1/1 -> Neural Network 1/1(X)
  Add3/1 -> [e1], [E2]
  [ti] -> Switch4/2
  Add11/1 -> Switch4/1
  Switch4/1 -> [ef]
  [P] -> n/1
  Un3/1 -> Sum10/1  "f"
  Sum10/1 -> Add23/2
  n/1 -> [MP1], Sum10/2
  [w1] -> Add23/1
  Add23/1 -> Switch4/3
  Add7/1 -> Integrator1/1
  Integrator4/1 -> [wt]
  Integrator1/1 -> [w1], f1/1, Integrator4/1
  Add5/1 -> [e2]
  [el] -> Gain8/1
  [S] -> Product16/2
  [Wl] -> Math Function2/1
  Math Function2/1 -> Product16/1
  Product16/1 -> Add21/2
  Gain8/1 -> Add21/1
  [Id] -> Add22/1
  [vd] -> Add22/2
  Add22/1 -> [el]
  [S] -> Product18/1
  Constant17/1 -> Product18/2
  [el] -> Product18/3
  Product18/1 -> Add24/1
  Constant18/1 -> Product17/1
  [Wl] -> Product17/2
  Product17/1 -> Add24/2
  Constant19/1 -> Product17/3
  Add24/1 -> Integrator5/1
  Integrator5/1 -> [Wl]
  Abs2/1 -> Product17/4
  [el] -> Abs2/1
  [vod] -> Add25/1
  Add25/1 -> [evd]
  Sum11/1 -> Add25/2
  [Q] -> m/1
  Un1/1 -> Sum11/2
  m/1 -> [NQ1], Sum11/1
  [evd] -> Gain9/1
  [S] -> Product19/2
  [Wv] -> Math Function4/1
  Math Function4/1 -> Product19/1
  Product19/1 -> Add20/2
  Gain9/1 -> Add20/1
  Add20/1 -> [vd]
  [S] -> Product21/1
  Constant20/1 -> Product21/2
  [evd] -> Product21/3
  Product21/1 -> Add26/1
  Constant21/1 -> Product20/1
  [Wl] -> Product20/2
  Product20/1 -> Add26/2
  Constant22/1 -> Product20/3
  Abs3/1 -> Product20/4
  [evd] -> Abs3/1
  Add26/1 -> Integrator6/1
  Integrator6/1 -> [Wv]
  [ti] -> Switch3/2
  Add8/1 -> Switch3/1
  Switch3/1 -> [vn1]
  Add21/1 -> Switch3/3
  Abs1/1 -> Product10/4
  [e2] -> Product8/3
  connections:
  C/RConn1 -- Ground1/LConn1 -- C/RConn3 -- C/RConn2
  L/RConn2 -- Three-Phase V-I Measurement1/LConn2 -- C/LConn2
  L/RConn1 -- Three-Phase V-I Measurement1/LConn1 -- C/LConn1
  L/RConn3 -- Three-Phase V-I Measurement1/LConn3 -- C/LConn3
  Controlled Voltage Source/LConn1 -- Controlled Voltage Source1/LConn1 -- Ground/LConn1 -- Controlled Voltage Source2/LConn1
  Three-Phase V-I Measurement/LConn1 -- Controlled Voltage Source/RConn1
  Controlled Voltage Source1/RConn1 -- Three-Phase V-I Measurement/LConn2
  Controlled Voltage Source2/RConn1 -- Three-Phase V-I Measurement/LConn3
  Three-Phase V-I Measurement/RConn1 -- L/LConn1
  Three-Phase V-I Measurement/RConn2 -- L/LConn2
  Three-Phase V-I Measurement/RConn3 -- L/LConn3
  Three-Phase V-I Measurement1/RConn1 -- Three-Phase Series RLC Branch4/RConn1
  Three-Phase V-I Measurement1/RConn2 -- Three-Phase Series RLC Branch4/RConn2
  Three-Phase V-I Measurement1/RConn3 -- Three-Phase Series RLC Branch4/RConn3
  Three-Phase Series RLC Branch4/LConn1 -- a/RConn1
  Three-Phase Series RLC Branch4/LConn2 -- b/RConn1
  Three-Phase Series RLC Branch4/LConn3 -- c/RConn1
